simulink model "Exercicio_1gball_sim"  (R2016a)
settings: Solver=VariableStepAuto  StartTime=0.0  StopTime=t_sim  RelTol=1e-3
values from neighbouring files (symbols this model uses):
  A_ball = [0 1 0 0 ... (first row only)    [Exercicio_2.m]
  AObs_ball = A_ball    [Exercicio_2.m]
  B_ball = [0;0;0;1]    [Exercicio_2.m]
  Ball_AObs = (Ball_Abb-(Ke_ball_ordmin*Ball_Aab))    [Exercicio_2.m]
  Ball_BObs = ((Ball_AObs*Ke_ball_ordmin) + Ball_Aba - (Ke_ball_ordmin*Ball_Aaa))    [Exercicio_2.m]
  Ball_CObs = [[0 0 0];[eye(3)]]    [Exercicio_2.m]
  Ball_DObs = [1;Ke_ball_ordmin]    [Exercicio_2.m]
  Ball_FObs = (Ball_Bb - (Ke_ball_ordmin*Ball_Ba))    [Exercicio_2.m]
  BObs_ball = B_ball    [Exercicio_2.m]
  C_ball = [1 0 0 0]    [Exercicio_2.m]
  CObs_ball = C_ball    [Exercicio_2.m]
  D_ball = [0]    [Exercicio_2.m]
  DObs_ball = D_ball    [Exercicio_2.m]
  K_ball = place(A_ball,B_ball,[p1_ball,p2_ball,p3_ball,p4_ball])    [Exercicio_2.m]
  Ke_ball = acker(AObs_ball,BObs_ball,pr_obs)    [Exercicio_2.m]
  N_termo = rscale(A_ball,B_ball,C_ball,D_ball,K_ball)    [Exercicio_2.m]
settings Model: Creator=Usuario  LastModifiedBy=Eletrônica Auto Poli

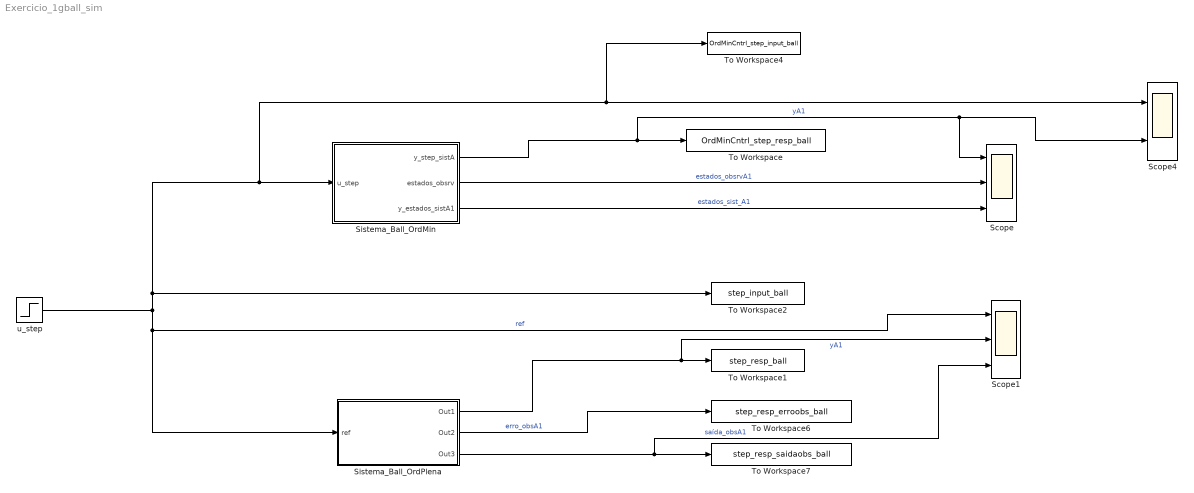
== system Exercicio_1gball_sim ==
  Scope : Scope  NumInputPorts=3
  Scope1 : Scope  NumInputPorts=3
  Scope4 : Scope  NumInputPorts=2
  Sistema_Ball_OrdMin : Subsystem
  Sistema_Ball_OrdPlena : Subsystem
  To Workspace : ToWorkspace  VariableName=OrdMinCntrl_step_resp_ball  SaveFormat=Timeseries  SampleTime=-1
  To Workspace1 : ToWorkspace  VariableName=step_resp_ball  SaveFormat=Timeseries  SampleTime=-1
  To Workspace2 : ToWorkspace  VariableName=step_input_ball  SaveFormat=Timeseries  SampleTime=-1
  To Workspace4 : ToWorkspace  VariableName=OrdMinCntrl_step_input_ball  SaveFormat=Timeseries  SampleTime=-1
  To Workspace6 : ToWorkspace  VariableName=step_resp_erroobs_ball  SaveFormat=Timeseries  SampleTime=-1
  To Workspace7 : ToWorkspace  VariableName=step_resp_saidaobs_ball  SaveFormat=Timeseries  SampleTime=-1
  u_step : Step  SampleTime=0.01
  wires:
  Sistema_Ball_OrdMin/1(y_step_sistA) -> Scope/1, Scope4/2, To Workspace/1  "yA1"
  Sistema_Ball_OrdMin/2(estados_obsrv) -> Scope/2  "estados_obsrvA1"
  Sistema_Ball_OrdMin/3(y_estados_sistA1) -> Scope/3  "estados_sist_A1"
  Sistema_Ball_OrdPlena/1(Out1) -> Scope1/2, To Workspace1/1  "yA1"
  Sistema_Ball_OrdPlena/2(Out2) -> To Workspace6/1  "erro_obsA1"
  Sistema_Ball_OrdPlena/3(Out3) -> Scope1/3, To Workspace7/1  "saída_obsA1"
  u_step/1 -> Sistema_Ball_OrdPlena/1(ref), Scope1/1, To Workspace2/1, To Workspace4/1, Scope4/1, Sistema_Ball_OrdMin/1(u_step)  "ref"

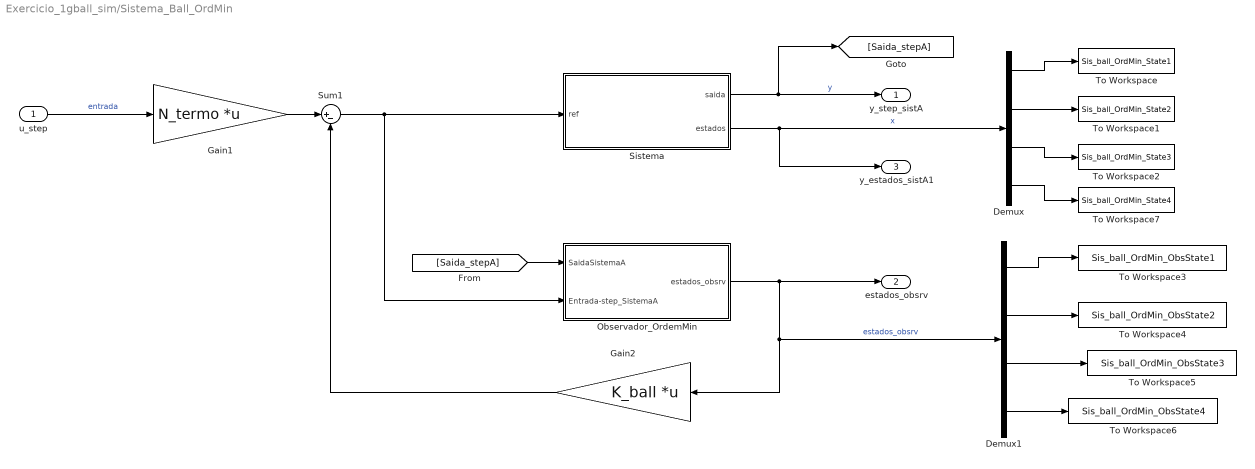
== system Exercicio_1gball_sim/Sistema_Ball_OrdMin ==
  u_step : Inport
  Demux : Demux
  Demux1 : Demux
  Gain1 : Gain  Gain=N_termo  Multiplication=Matrix(K*u)
  Gain2 : Gain  Gain=K_ball  Multiplication=Matrix(K*u)
  Observador_OrdemMin : Subsystem
  Sistema : Subsystem
  Sum1 : Sum  Inputs=|+-
  To Workspace : ToWorkspace  VariableName=Sis_ball_OrdMin_State1  SaveFormat=Timeseries  SampleTime=-1
  To Workspace1 : ToWorkspace  VariableName=Sis_ball_OrdMin_State2  SaveFormat=Timeseries  SampleTime=-1
  To Workspace2 : ToWorkspace  VariableName=Sis_ball_OrdMin_State3  SaveFormat=Timeseries  SampleTime=-1
  To Workspace3 : ToWorkspace  VariableName=Sis_ball_OrdMin_ObsState1  SaveFormat=Timeseries  SampleTime=-1
  To Workspace4 : ToWorkspace  VariableName=Sis_ball_OrdMin_ObsState2  SaveFormat=Timeseries  SampleTime=-1
  To Workspace5 : ToWorkspace  VariableName=Sis_ball_OrdMin_ObsState3  SaveFormat=Timeseries  SampleTime=-1
  To Workspace6 : ToWorkspace  VariableName=Sis_ball_OrdMin_ObsState4  SaveFormat=Timeseries  SampleTime=-1
  To Workspace7 : ToWorkspace  VariableName=Sis_ball_OrdMin_State4  SaveFormat=Timeseries  SampleTime=-1
  y_step_sistA : Outport
  estados_obsrv : Outport  Port=2
  y_estados_sistA1 : Outport  Port=3
  wires:
  Demux/1 -> To Workspace/1
  Demux/2 -> To Workspace1/1
  Demux/3 -> To Workspace2/1
  Sistema/1(saida) -> [Saida_stepA], y_step_sistA/1  "y"
  Sistema/2(estados) -> y_estados_sistA1/1, Demux/1  "x"
  Demux1/1 -> To Workspace3/1
  Demux1/2 -> To Workspace4/1
  Observador_OrdemMin/1(estados_obsrv) -> Gain2/1, Demux1/1, estados_obsrv/1  "estados_obsrv"
  [Saida_stepA] -> Observador_OrdemMin/1(SaidaSistemaA)
  Demux1/3 -> To Workspace5/1
  Demux1/4 -> To Workspace6/1
  Demux/4 -> To Workspace7/1
  Sum1/1 -> Observador_OrdemMin/2(Entrada-step_SistemaA), Sistema/1(ref)
  Gain2/1 -> Sum1/2
  Gain1/1 -> Sum1/1
  u_step/1 -> Gain1/1  "entrada"

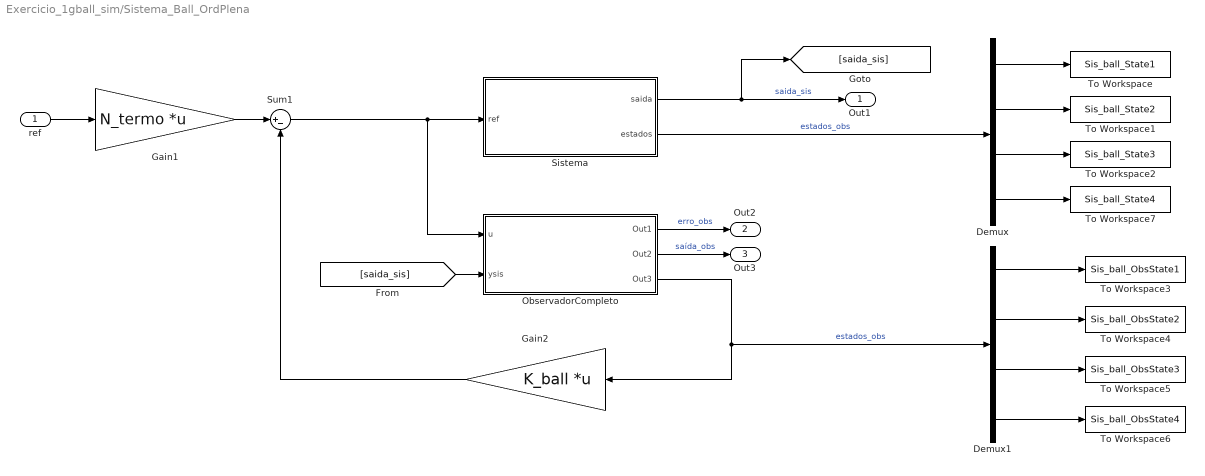
== system Exercicio_1gball_sim/Sistema_Ball_OrdPlena ==
  ref : Inport
  Demux : Demux
  Demux1 : Demux
  Gain1 : Gain  Gain=N_termo  Multiplication=Matrix(K*u)
  Gain2 : Gain  Gain=K_ball  Multiplication=Matrix(K*u)
  ObservadorCompleto : Subsystem
  Sistema : Subsystem
  Sum1 : Sum  Inputs=|+-
  To Workspace : ToWorkspace  VariableName=Sis_ball_State1  SaveFormat=Timeseries  SampleTime=-1
  To Workspace1 : ToWorkspace  VariableName=Sis_ball_State2  SaveFormat=Timeseries  SampleTime=-1
  To Workspace2 : ToWorkspace  VariableName=Sis_ball_State3  SaveFormat=Timeseries  SampleTime=-1
  To Workspace3 : ToWorkspace  VariableName=Sis_ball_ObsState1  SaveFormat=Timeseries  SampleTime=-1
  To Workspace4 : ToWorkspace  VariableName=Sis_ball_ObsState2  SaveFormat=Timeseries  SampleTime=-1
  To Workspace5 : ToWorkspace  VariableName=Sis_ball_ObsState3  SaveFormat=Timeseries  SampleTime=-1
  To Workspace6 : ToWorkspace  VariableName=Sis_ball_ObsState4  SaveFormat=Timeseries  SampleTime=-1
  To Workspace7 : ToWorkspace  VariableName=Sis_ball_State4  SaveFormat=Timeseries  SampleTime=-1
  Out1 : Outport
  Out2 : Outport  Port=2
  Out3 : Outport  Port=3
  wires:
  Demux/1 -> To Workspace/1
  Demux/2 -> To Workspace1/1
  Demux/3 -> To Workspace2/1
  Demux1/1 -> To Workspace3/1
  Demux1/2 -> To Workspace4/1
  Demux1/3 -> To Workspace5/1
  ObservadorCompleto/1(Out1) -> Out2/1  "erro_obs"
  ObservadorCompleto/2(Out2) -> Out3/1  "saída_obs"
  Demux1/4 -> To Workspace6/1
  Demux/4 -> To Workspace7/1
  Sum1/1 -> Sistema/1(ref), ObservadorCompleto/1(u)
  Gain2/1 -> Sum1/2
  Gain1/1 -> Sum1/1
  ref/1 -> Gain1/1
  Sistema/2(estados) -> Demux/1  "estados_obs"
  ObservadorCompleto/3(Out3) -> Demux1/1, Gain2/1  "estados_obs"
  Sistema/1(saida) -> Out1/1, [saida_sis]  "saida_sis"
  [saida_sis] -> ObservadorCompleto/2(ysis)

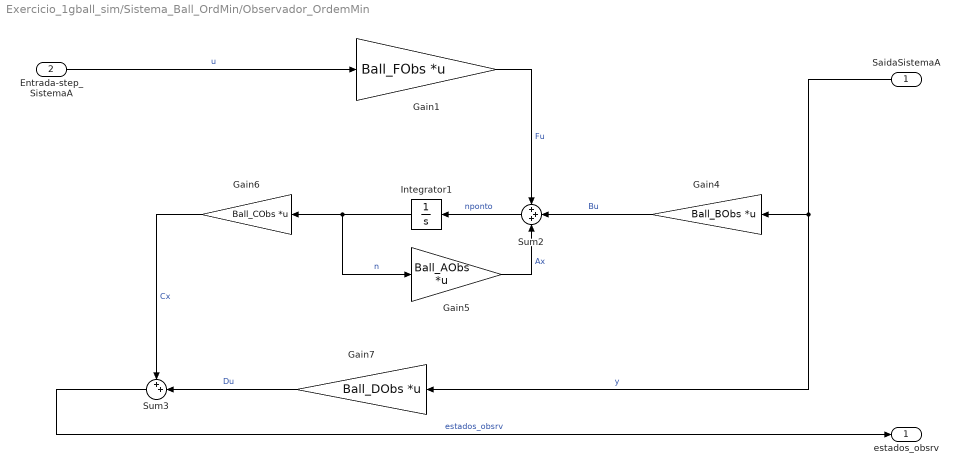
== system Exercicio_1gball_sim/Sistema_Ball_OrdMin/Observador_OrdemMin ==
  SaidaSistemaA : Inport
  Entrada-step_SistemaA : Inport  Port=2
  Gain1 : Gain  Gain=Ball_FObs  Multiplication=Matrix(K*u)
  Gain4 : Gain  Gain=Ball_BObs  Multiplication=Matrix(K*u)
  Gain5 : Gain  Gain=Ball_AObs  Multiplication=Matrix(K*u)
  Gain6 : Gain  Gain=Ball_CObs  Multiplication=Matrix(K*u)
  Gain7 : Gain  Gain=Ball_DObs  Multiplication=Matrix(K*u)
  Integrator1 : Integrator  InitialCondition=[1 3 2]  UpperSaturationLimit=1.279387983436996e+55  LowerSaturationLimit=0
  Sum2 : Sum  Inputs=+++
  Sum3 : Sum  Inputs=++|
  estados_obsrv : Outport
  wires:
  Integrator1/1 -> Gain5/1, Gain6/1  "n"
  Gain6/1 -> Sum3/1  "Cx"
  SaidaSistemaA/1 -> Gain4/1, Gain7/1  "y"
  Sum3/1 -> estados_obsrv/1  "estados_obsrv"
  Gain7/1 -> Sum3/2  "Du"
  Gain4/1 -> Sum2/2  "Bu"
  Gain5/1 -> Sum2/3  "Ax"
  Gain1/1 -> Sum2/1  "Fu"
  Sum2/1 -> Integrator1/1  "nponto"
  Entrada-step_SistemaA/1 -> Gain1/1  "u"

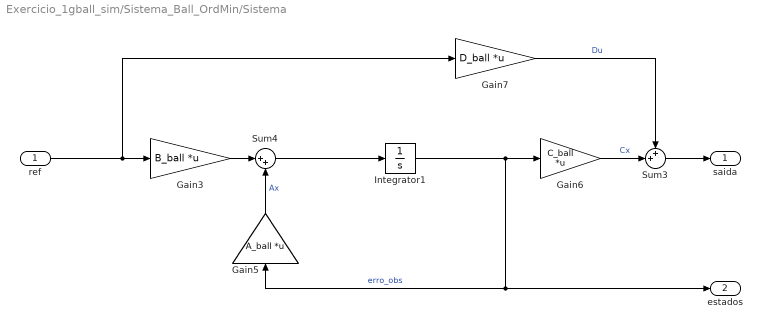
== system Exercicio_1gball_sim/Sistema_Ball_OrdMin/Sistema ==
  ref : Inport
  Gain3 : Gain  Gain=B_ball  Multiplication=Matrix(K*u)
  Gain5 : Gain  Gain=A_ball  Multiplication=Matrix(K*u)
  Gain6 : Gain  Gain=C_ball  Multiplication=Matrix(K*u)
  Gain7 : Gain  Gain=D_ball  Multiplication=Matrix(K*u)
  Integrator1 : Integrator
  Sum3 : Sum  Inputs=++|
  Sum4 : Sum  Inputs=|++
  saida : Outport
  estados : Outport  Port=2
  wires:
  Gain6/1 -> Sum3/2  "Cx"
  Gain5/1 -> Sum4/2  "Ax"
  Sum4/1 -> Integrator1/1
  Integrator1/1 -> estados/1, Gain5/1, Gain6/1  "erro_obs"
  Gain3/1 -> Sum4/1
  Gain7/1 -> Sum3/1  "Du"
  Sum3/1 -> saida/1
  ref/1 -> Gain7/1, Gain3/1

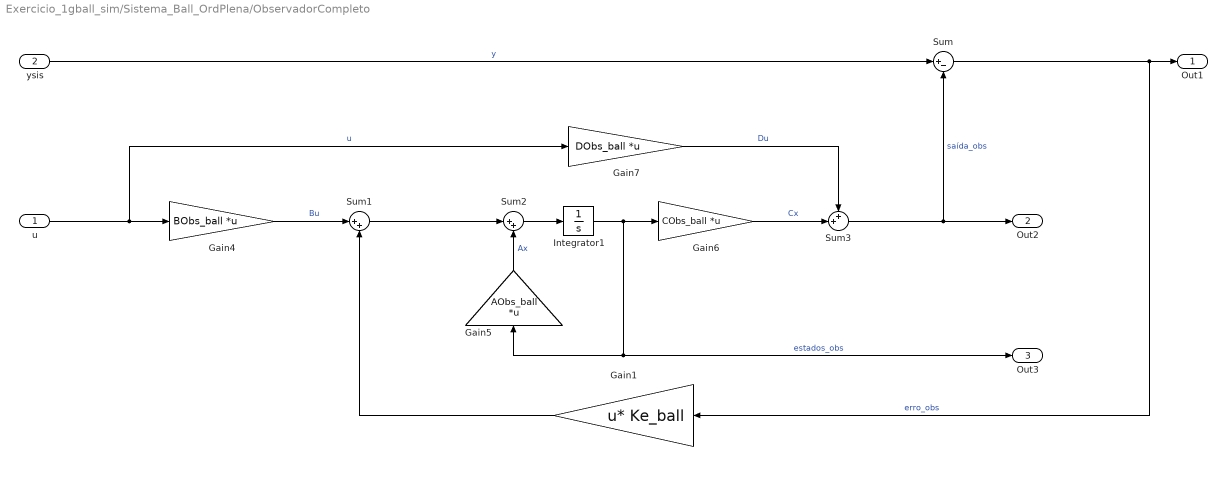
== system Exercicio_1gball_sim/Sistema_Ball_OrdPlena/ObservadorCompleto ==
  u : Inport
  ysis : Inport  Port=2
  Gain1 : Gain  Gain=Ke_ball  Multiplication=Matrix(u*K)
  Gain4 : Gain  Gain=BObs_ball  Multiplication=Matrix(K*u)
  Gain5 : Gain  Gain=AObs_ball  Multiplication=Matrix(K*u)
  Gain6 : Gain  Gain=CObs_ball  Multiplication=Matrix(K*u)
  Gain7 : Gain  Gain=DObs_ball  Multiplication=Matrix(K*u)
  Integrator1 : Integrator  InitialCondition=[1 3 1 2]
  Sum : Sum  Inputs=|+-
  Sum1 : Sum  Inputs=|++
  Sum2 : Sum  Inputs=|++
  Sum3 : Sum  Inputs=++|
  Out1 : Outport
  Out2 : Outport  Port=2
  Out3 : Outport  Port=3
  wires:
  Sum3/1 -> Out2/1, Sum/2  "saída_obs"
  Integrator1/1 -> Out3/1, Gain5/1, Gain6/1  "estados_obs"
  Gain6/1 -> Sum3/2  "Cx"
  Gain7/1 -> Sum3/1  "Du"
  Gain4/1 -> Sum1/1  "Bu"
  Gain5/1 -> Sum2/2  "Ax"
  Sum2/1 -> Integrator1/1
  ysis/1 -> Sum/1  "y"
  u/1 -> Gain4/1, Gain7/1  "u"
  Sum/1 -> Out1/1, Gain1/1  "erro_obs"
  Sum1/1 -> Sum2/1
  Gain1/1 -> Sum1/2

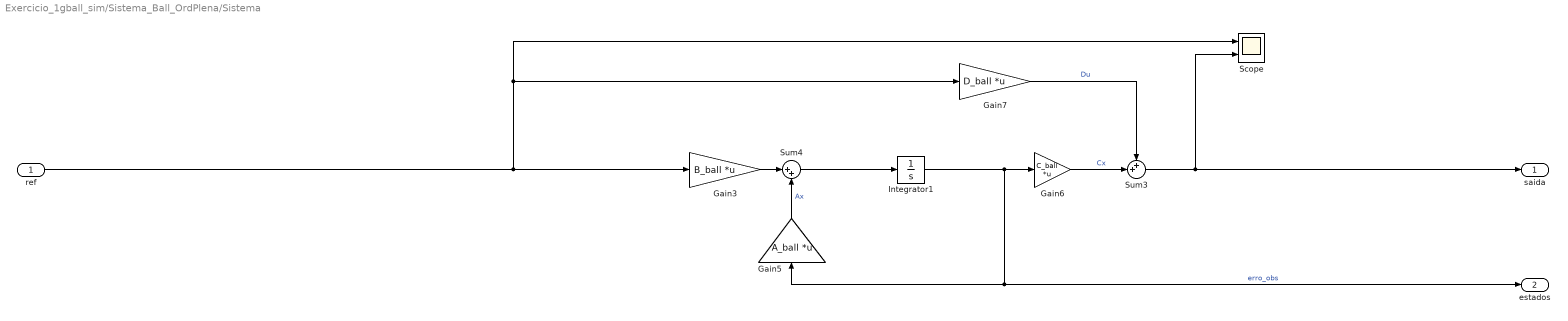
== system Exercicio_1gball_sim/Sistema_Ball_OrdPlena/Sistema ==
  ref : Inport
  Gain3 : Gain  Gain=B_ball  Multiplication=Matrix(K*u)
  Gain5 : Gain  Gain=A_ball  Multiplication=Matrix(K*u)
  Gain6 : Gain  Gain=C_ball  Multiplication=Matrix(K*u)
  Gain7 : Gain  Gain=D_ball  Multiplication=Matrix(K*u)
  Integrator1 : Integrator
  Scope : Scope  NumInputPorts=2
  Sum3 : Sum  Inputs=++|
  Sum4 : Sum  Inputs=|++
  saida : Outport
  estados : Outport  Port=2
  wires:
  Gain6/1 -> Sum3/2  "Cx"
  Gain5/1 -> Sum4/2  "Ax"
  Sum4/1 -> Integrator1/1
  Integrator1/1 -> estados/1, Gain5/1, Gain6/1  "erro_obs"
  Gain3/1 -> Sum4/1
  Gain7/1 -> Sum3/1  "Du"
  Sum3/1 -> Scope/2, saida/1
  ref/1 -> Gain7/1, Scope/1, Gain3/1
